simulink model "Model_15_11062020_3_Lev_Unbalance_SVM_AB21"  (R2021a)
settings: Solver=FixedStepAuto  StartTime=0.0  StopTime=0.03  FixedStep=Ts/10  MaxStep=1e-4  RelTol=1e-3
InitFcn:
  | Ts=1/(12000);
  | Ts_Control=Ts;
  | Ts_Power=Ts;
  | PulseDuration=5e-6;
  | Vrefpeak=399;
  | VDC=800;
  | R=1.4;
  | L=1e-4;
  | Freq = 120;
  | Rc= 0.00001;
  | C=220e-6;
  | Ld = 473e-6;
  | Lq = 1155e-6;
  | Fpm = 0.1383;
  | Rs = 0.036;
  | 
  | 
  | %%%%%Switch Characterization START%%%%%
  | T003_Thermal_Initialization;
  | T020_Characterizing_SKiM401MLI07E4_Simulink_Model_v1_0;
  | %%%%%Switch Characterization END%%%%%%
undefined symbols (not defined in the file or in its folder): Cond_Loss_Diode, Cond_Loss_IGBT, Page_Temp_C, Reverse_Rec_Diode, TurnoffIGBT, TurnonIGBT
libraries: spsMeanLib x35, simulink x28, spsMonostableLib x14, spsSampleandHoldLib x14, spsIGBTDiodeLib x12, spsDiodeLib x6, spsCurrentMeasurementLib x4, spsFirstOrderFilterLib x3, spsSeriesRLCBranchLib x3, spsVoltageMeasurementLib x3, pid_lib x2, spsAlphaBetaZerotoabcLib x1
(part 1 of 2)
settings Model: Creator=seoga  LastModifiedBy=Monster
settings SolverCC: AlgebraicLoopSolver=TrustRegion
settings DataIOCC: ReturnWorkspaceOutputs=off
settings DebuggingCC: SFMachineParentedDataDiag=warning  ArithmeticOperatorsInVariantConditions=warning
settings SFSimCC: SimUseLocalCustomCode=off  CustomCodeUndefinedFunction=UseInterfaceOnly
settings RTWCC: RTWUseLocalCustomCode=off

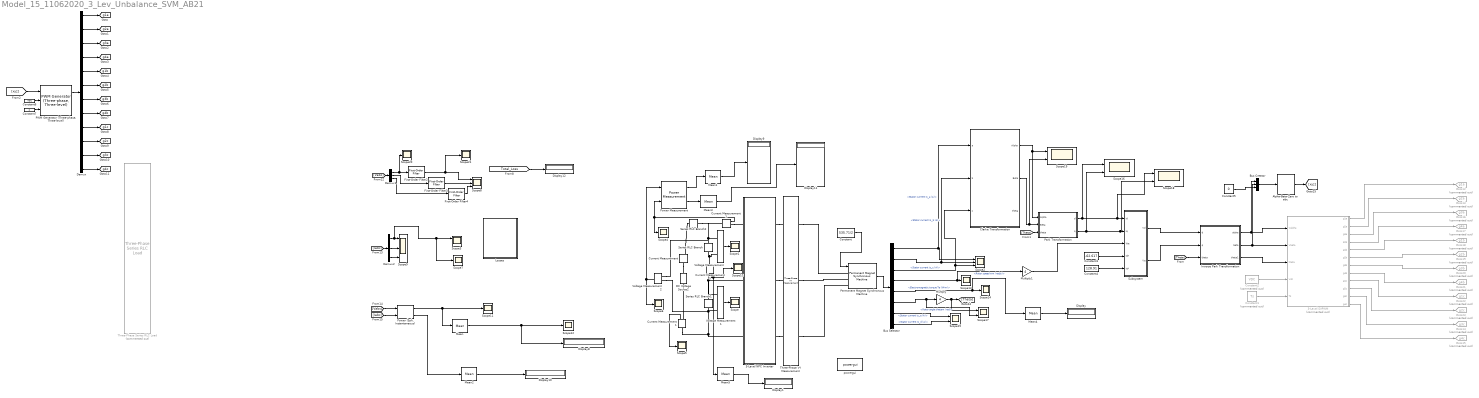
== system Model_15_11062020_3_Lev_Unbalance_SVM_AB21 ==
  3-Level NPC Inverter : Subsystem
  3-Level SVPWM : Subsystem  Commented=on
  Alpha-Beta-Zero to abc : spsAlphaBetaZerotoabcLib/Alpha-Beta-Zero to abc
      settings: SourceProductBaseCode=PS
  Bus Creator : BusCreator  Inputs=3
  Bus Selector : BusSelector  OutputSignals=Stator current is_a (A),Stator current is_b (A),Stator current is_c (A),Rotor speed wm (rad/s),Electromagnetic torque Te (N*m),Rotor angle thetam (rad),Stator current is_q (A),Stator current is_d (A)
  Clarke Transformation : Subsystem
  Constant : Constant  Value=535.71/2
  Constant1 : Constant  Commented=on  Value=Ts
  Constant2 : Constant  Commented=on  Value=VDC
  Constant3 : Constant  Value=-62.617
  Constant4 : Constant  Value=128.91
  Constant5 : Constant  Value=0
  Constant6 : Constant  Value=VDC
  Constant7 : Constant  Value=0
  Current Measurement{,1..3} (4 alike) : spsCurrentMeasurementLib/Current Measurement  PhasorSimulation=off  OutputType=Complex  PSBequivalent=0
  DC Voltage Source2 : spsDCVoltageSourceLib/DC Voltage Source  Amplitude=VDC  Measurements=None
  Demux : Demux  Outputs=12
  Demux1 : Demux  Outputs=3
  Demux2 : Demux  Outputs=3
  Display{,1,8..12} (7 alike) : Display
  First-Order Filter2 : spsFirstOrderFilterLib/First-Order Filter  FilterType=Lowpass  Tc=1e-4*2.5  Ts=0  Initialize=on  Vac_Init=[0, 0, 350/4]  Vdc_Init=0  PlotResponse=off  FreqRange="[0,  200,  1]"
  First-Order Filter3 : spsFirstOrderFilterLib/First-Order Filter  FilterType=Lowpass  Tc=1e-4  Ts=0  Initialize=on  Vac_Init=[0, 0, 350]  Vdc_Init=0  PlotResponse=off  FreqRange="[0,  200,  1]"
  First-Order Filter4 : spsFirstOrderFilterLib/First-Order Filter  FilterType=Lowpass  Tc=1e-4  Ts=0  Initialize=on  Vac_Init=[0, 0, 350]  Vdc_Init=0  PlotResponse=off  FreqRange="[0,  200,  1]"
  Goto12 : Goto  Commented=on  GotoTag=g1a  TagVisibility=global
  Goto13 : Goto  Commented=on  GotoTag=g2a  TagVisibility=global
  Goto14 : Goto  Commented=on  GotoTag=g3c  TagVisibility=global
  Goto15 : Goto  Commented=on  GotoTag=g4c  TagVisibility=global
  Goto16 : Goto  Commented=on  GotoTag=g3a  TagVisibility=global
  Goto17 : Goto  Commented=on  GotoTag=g4a  TagVisibility=global
  Goto18 : Goto  Commented=on  GotoTag=g1b  TagVisibility=global
  Goto19 : Goto  Commented=on  GotoTag=g2b  TagVisibility=global
  Goto20 : Goto  Commented=on  GotoTag=g3b  TagVisibility=global
  Goto21 : Goto  Commented=on  GotoTag=g4b  TagVisibility=global
  Goto22 : Goto  Commented=on  GotoTag=g1c  TagVisibility=global
  Goto23 : Goto  Commented=on  GotoTag=g2c  TagVisibility=global
  Inverse Park Transformation : Subsystem
  Losses : Subsystem
  Mean{,1..3} (4 alike) : spsMeanLib/Mean  Freq=Freq  Vinit=0  Ts=0
  Mean4 : spsMeanLib/Mean  Freq=1200  Vinit=0  Ts=0
  Mean5 : spsMeanLib/Mean  Freq=10  Vinit=0  Ts=0
  Multiply : Gain  Gain=4
  Multiply1 : Gain  Gain=4
  "PWM Generator (Three-phase, Three-level)" : eePwmGeneratorThreeLevel/PWM Generator (Three-phase, Three-level)  CPWMMode=SVM: space vector modulation  fsw=1/Ts  Ts=Ts/10
      settings: SourceProductBaseCode=PS  SamplingMode=Natural
  Park Transformation : Subsystem
  Permanent Magnet Synchronous Machine : spsPermanentMagnetSynchronousMachineLib/Permanent Magnet Synchronous Machine  NbPhases=3  FluxDistribution=Sinusoidal  RotorType=Salient-pole  MechanicalLoad=Speed w  PresetModel=No  ShowDetailedParameters=on  MeasurementBus=off  Resistance=0.036  Inductance=8.5e-3  dqInductances=[0.473e-3,1.155e-3]  La=0.000395  MachineConstant=Flux linkage established by magnets (V.s)  Flux=0.1383  VoltageCst=100.3394  TorqueCst=0.8298  Flat=120  Mechanical=[0.0027 0.0004924 4 0]  PolePairs=4  InitialConditions=[0,0, 0,0]  InitialConditions5ph=[0 0 0 0 0 0]  RefAngle=Aligned with phase A axis (original Park)  IterativeDiscreteModel=Trapezoidal non iterative  TsBlock=-1  TsPowergui=0
  "Power (3ph, Instantaneous)" : spsPower3phInstantaneousLib/Power (3ph, Instantaneous)
  Power Measurement : eePowerMeasurement/Power Measurement  LabelModeActiveChoice=Continuous  F=60  K=[0 1 2 3]  Ts=0
      settings: SourceProductBaseCode=PS
  Scope{,1,4..7,10..14,20..21} (13 alike) : Scope
  Scope{3,15..19} (6 alike) : Scope  NumInputPorts=2
  Scope2 : Scope  NumInputPorts=3
  Scope8 : Scope  NumInputPorts=3
  Scope9 : Scope  NumInputPorts=3
  Series RLC Branch : spsSeriesRLCBranchLib/Series RLC Branch  LConnTagsString=__new0  RConnTagsString=__new0  BranchType=RC  Resistance=Rc  Inductance=1e-3  SetiL0=off  InitialCurrent=0  Capacitance=C  Setx0=on  InitialVoltage=VDC/2  Measurements=None
  Series RLC Branch1 : spsSeriesRLCBranchLib/Series RLC Branch  LConnTagsString=__new0  RConnTagsString=__new0  BranchType=RC  Resistance=Rc  Inductance=1e-3  SetiL0=off  InitialCurrent=0  Capacitance=C  Setx0=on  InitialVoltage=VDC/2  Measurements=None
  Series RLC Branch2 : spsSeriesRLCBranchLib/Series RLC Branch  LConnTagsString=__new0  RConnTagsString=__new0  BranchType=R  Resistance=1e-6  Inductance=1e-3  SetiL0=off  InitialCurrent=0  Capacitance=470e-6  Setx0=on  InitialVoltage=400  Measurements=None
  Subsystem : Subsystem
  Three-Phase Series RLC Load : spsThreePhaseSeriesRLCLoadLib/Three-Phase Series RLC Load  Commented=on  LConnTagsString=A|B|C  Configuration=Y (grounded)  NominalVoltage=Vrefpeak*sqrt(3/2)  Vabc=[1e3 1e3 1e3]  Vabcp=[1e3 1e3 1e3]  NominalFrequency=Freq  UnbalancedPower=off  ActivePower=150e3  InductivePower=100e3  CapacitivePower=0  Pabc=[10e3 9e3 11e3]  QLabc=[100 90 110]  QCabc=[100 90 110]  Pabcp=[10e3 9e3 11e3]  QLabcp=[100 90 110]  QCabcp=[100 90 110]  Measurements=None  LoadType=constant Z
  Three-Phase V-I Measurement : spsThreePhaseVIMeasurementLib/Three-Phase V-I Measurement  VoltageMeasurement=phase-to-phase  SetLabelV=on  LabelV=Vabc  Vpu=off  VpuLL=off  CurrentMeasurement=yes  SetLabelI=on  LabelI=Iabc  Ipu=off  Pbase=100e6  Vbase=500e3  OutputType=Complex  PhasorSimulation=off  PSBequivalent=0
  Voltage Measurement : spsVoltageMeasurementLib/Voltage Measurement  PhasorSimulation=off  OutputType=Complex  PSBequivalent=0
  Voltage Measurement1 : spsVoltageMeasurementLib/Voltage Measurement  PhasorSimulation=off  OutputType=Complex  PSBequivalent=0
  Voltage Measurement2 : spsVoltageMeasurementLib/Voltage Measurement  PhasorSimulation=off  OutputType=Complex  PSBequivalent=0
  powergui : spspowerguiLib/powergui  Priority=1  SimulationMode=Discrete  SampleTime=Ts/10  frequency=60  Iterations=50  frequencyindice=0  Pbase=100e6  ErrMax=1e-4  UnitsV=kV  UnitsW=MW  buscounter=0  FunctionMessages=off  echomessages=off  EnableUseOfTLC=off  CurrentSourceSwitches=off  DisableSnubberDevices=off  DisableRonSwitches=off  DisableVfSwitches=off  DisplayEquations=off  AutomaticDiscreteSolvers=off  SolverType=Tustin/Backward Euler (TBE)  Interpol=off  ExternalGateDelay=off  methode=off  Ts=100  x0status=blocks  SPID=off  SwTol=0  HookPort=off  NonlinearTolerance=1e-4  nMaxIteration=100  ContinueOnMaxIteration=off  RestoreLinks=warning  ResistiveCurrentMeasurement=off  Frange=[0:2:500]  Ylog=off  Xlog=on  ShowGrid=off  save=off  variable=ZData  structure=0  ZoomFFT=off  StartTime=0.0  cycles=1  DisplayStyle=1  fundamental=60  FreqAxis=off  MaxFrequency=1000  frequencyindicesteady=1  RmsSteady=1  display=off
  tag scope: g1a=global, g1b=global, g1c=global, g2a=global, g2b=global, g2c=global, g3a=global, g3b=global, g3c=global, g4a=global, g4b=global, g4c=global
  wires:
  Bus Selector/2 -> Clarke Transformation/2(b), Scope2/2  "<Stator current is_b (A)>"
  Demux1/3 -> First-Order Filter4/1
  "Power (3ph, Instantaneous)"/1 -> Mean/1, Scope11/1
  [Vabc] -> Demux1/1
  Demux1/2 -> First-Order Filter3/1
  First-Order Filter4/1 -> Scope8/3
  [Vabc] -> "Power (3ph, Instantaneous)"/1
  Demux1/1 -> Scope20/1, First-Order Filter2/1
  [Iabc] -> Demux2/1
  [Iabc] -> "Power (3ph, Instantaneous)"/2
  First-Order Filter3/1 -> Scope8/2
  Voltage Measurement1/1 -> Scope/1
  Voltage Measurement/1 -> Scope1/1
  Constant7/1 -> "PWM Generator (Three-phase, Three-level)"/3
  Constant6/1 -> "PWM Generator (Three-phase, Three-level)"/2
  Demux/10 -> [g2c]
  Demux/3 -> [g3a]
  Demux/4 -> [g4a]
  Demux/7 -> [g3b]
  Demux/8 -> [g4b]
  Demux/5 -> [g1b]
  Demux/11 -> [g3c]
  Demux/6 -> [g2b]
  "PWM Generator (Three-phase, Three-level)"/1 -> Demux/1
  Demux/1 -> [g1a]
  Demux/2 -> [g2a]
  Demux/9 -> [g1c]
  Demux/12 -> [g4c]
  Mean/1 -> Display8/1, Scope12/1
  Mean2/1 -> Display10/1
  "Power (3ph, Instantaneous)"/2 -> Mean2/1
  Demux2/1 -> Scope7/1, Scope3/1, Scope9/1
  Demux2/2 -> Scope9/2
  Demux2/3 -> Scope9/3
  Voltage Measurement2/1 -> Scope6/1, Power Measurement/1
  Power Measurement/1 -> Mean1/1
  Mean1/1 -> Display9/1
  Power Measurement/2 -> Mean3/1
  Mean3/1 -> Display11/1
  Current Measurement1/1 -> Scope5/1
  Current Measurement2/1 -> Scope4/1, Power Measurement/2
  [Total_Loss] -> Display12/1
  Current Measurement3/1 -> Mean5/1, Scope10/1
  Permanent Magnet Synchronous Machine/1 -> Bus Selector/1
  3-Level SVPWM/2(g2a) -> Goto13/1
  3-Level SVPWM/1(g1a) -> Goto12/1
  3-Level SVPWM/11(g3c) -> Goto14/1
  3-Level SVPWM/6(g2b) -> Goto19/1
  3-Level SVPWM/4(g4a) -> Goto17/1
  3-Level SVPWM/8(g4b) -> Goto21/1
  3-Level SVPWM/9(g1c) -> Goto22/1
  3-Level SVPWM/10(g2c) -> Goto23/1
  3-Level SVPWM/7(g3b) -> Goto20/1
  3-Level SVPWM/12(g4c) -> Goto15/1
  3-Level SVPWM/3(g3a) -> Goto16/1
  3-Level SVPWM/5(g1b) -> Goto18/1
  Inverse Park Transformation/1(alpha) -> Bus Creator/1, 3-Level SVPWM/1(Valpha)
  Inverse Park Transformation/2(beta) -> Bus Creator/2, 3-Level SVPWM/2(Vbeta)
  Inverse Park Transformation/3(theta1) -> 3-Level SVPWM/3(theta)
  Constant1/1 -> 3-Level SVPWM/5(Ts)
  Constant2/1 -> 3-Level SVPWM/4(Vdc)
  Bus Selector/1 -> Clarke Transformation/1(a), Scope2/1  "<Stator current is_a (A)>"
  Bus Selector/3 -> Clarke Transformation/3(c), Scope2/3  "<Stator current is_c (A)>"
  Bus Selector/4 -> Multiply1/1, Scope13/1  "<Rotor speed wm (rad/s)>"
  Bus Selector/5 -> Mean4/1, Scope14/1  "<Electromagnetic torque Te (N*m)>"
  Constant/1 -> Permanent Magnet Synchronous Machine/1
  [Theta] -> Inverse Park Transformation/3(theta)
  Clarke Transformation/1(Alpha) -> Scope19/1, Park Transformation/1(Alpha)
  Clarke Transformation/2(Beta) -> Scope19/2, Park Transformation/2(Beta)
  [Theta] -> Park Transformation/3(theta)
  Bus Selector/6 -> Scope17/2, Multiply/1  "<Rotor angle thetam (rad)>"
  Multiply/1 -> Scope17/1, [Theta]
  Multiply1/1 -> Subsystem/3(We)
  Constant4/1 -> Subsystem/5(Iq*)
  Constant3/1 -> Subsystem/4(Id*)
  Subsystem/2(Vq) -> Inverse Park Transformation/2(q)
  Subsystem/1(Vd) -> Inverse Park Transformation/1(d)
  Bus Selector/7 -> Scope15/1  "<Stator current is_q (A)>"
  Bus Selector/8 -> Scope15/2  "<Stator current is_d (A)>"
  Mean4/1 -> Display/1
  Mean5/1 -> Display1/1
  Park Transformation/1(d) -> Scope18/1, Subsystem/1(Id), Scope16/1
  Park Transformation/2(q) -> Scope18/2, Subsystem/2(Iq), Scope16/2
  Bus Creator/1 -> Alpha-Beta-Zero to abc/1
  [xyz] -> "PWM Generator (Three-phase, Three-level)"/1
  Alpha-Beta-Zero to abc/1 -> [xyz]
  Constant5/1 -> Bus Creator/3
  First-Order Filter2/1 -> Scope21/1, Scope8/1
  connections:
  Series RLC Branch/LConn1 -- Series RLC Branch2/RConn1 -- Current Measurement2/LConn1 -- Voltage Measurement2/LConn1 -- Voltage Measurement/LConn1
  Series RLC Branch/RConn1 -- Current Measurement3/LConn1 -- Voltage Measurement/LConn2
  Series RLC Branch1/RConn1 -- Voltage Measurement2/LConn2 -- Voltage Measurement1/LConn2 -- Current Measurement1/LConn1 -- 3-Level NPC Inverter/LConn3
  Current Measurement/RConn1 -- Series RLC Branch2/LConn1
  Current Measurement/LConn1 -- DC Voltage Source2/RConn1
  Current Measurement1/RConn1 -- DC Voltage Source2/LConn1
  Current Measurement2/RConn1 -- 3-Level NPC Inverter/LConn1
  Series RLC Branch1/LConn1 -- Voltage Measurement1/LConn1 -- Current Measurement3/RConn1 -- 3-Level NPC Inverter/LConn2
  3-Level NPC Inverter/RConn1 -- Three-Phase V-I Measurement/LConn1
  Three-Phase V-I Measurement/RConn1 -- Permanent Magnet Synchronous Machine/LConn1
  Three-Phase V-I Measurement/RConn2 -- Permanent Magnet Synchronous Machine/LConn2
  3-Level NPC Inverter/RConn2 -- Three-Phase V-I Measurement/LConn2
  Three-Phase V-I Measurement/RConn3 -- Permanent Magnet Synchronous Machine/LConn3
  3-Level NPC Inverter/RConn3 -- Three-Phase V-I Measurement/LConn3

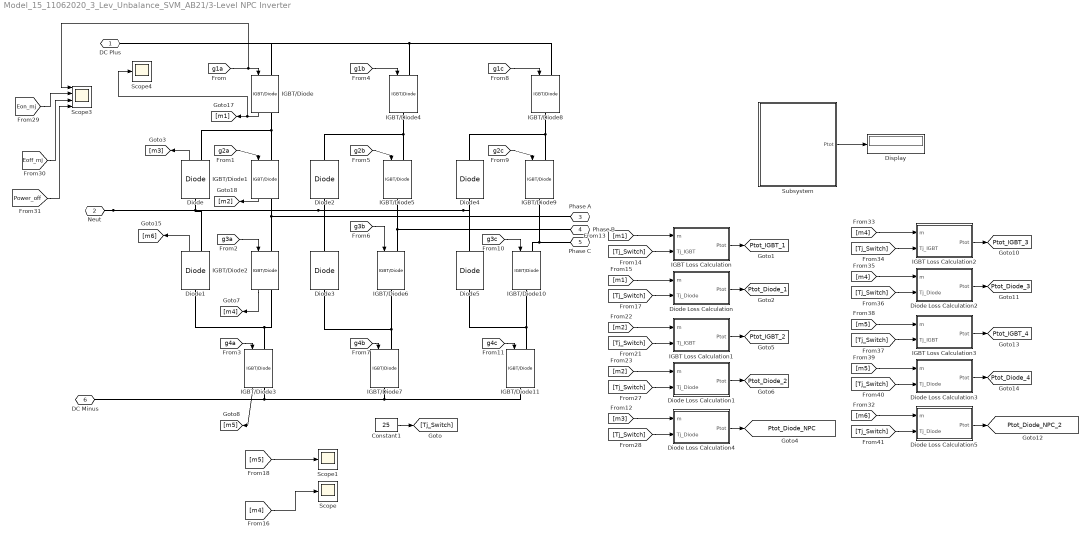
== system Model_15_11062020_3_Lev_Unbalance_SVM_AB21/3-Level NPC Inverter ==
  Constant1 : Constant  Value=25
  Diode : spsDiodeLib/Diode  Ron=1e-5  Lon=0  Vf=0.8  IC=0  UseSnubber=0  Rs=1e6  Cs=inf  Measurements=on
  Diode Loss Calculation : Subsystem
  Diode Loss Calculation1 : Subsystem
  Diode Loss Calculation2 : Subsystem
  Diode Loss Calculation3 : Subsystem
  Diode Loss Calculation4 : Subsystem
  Diode Loss Calculation5 : Subsystem
  Diode1 : spsDiodeLib/Diode  Ron=1e-5  Lon=0  Vf=0.8  IC=0  UseSnubber=0  Rs=1e6  Cs=inf  Measurements=on
  Diode{2..5} (4 alike) : spsDiodeLib/Diode  Ron=1e-5  Lon=0  Vf=0.8  IC=0  UseSnubber=0  Rs=1e6  Cs=inf  Measurements=off
  Display : Display
  IGBT Loss Calculation : Subsystem
  IGBT Loss Calculation1 : Subsystem
  IGBT Loss Calculation2 : Subsystem
  IGBT Loss Calculation3 : Subsystem
  IGBT/Diode{,1..3} (4 alike) : spsIGBTDiodeLib/IGBT//Diode  Ron=1e-3  Rs=1e6  Cs=inf  Measurements=on
  IGBT/Diode{4..11} (8 alike) : spsIGBTDiodeLib/IGBT//Diode  Ron=1e-3  Rs=1e6  Cs=inf  Measurements=off
  Scope : Scope
  Scope1 : Scope
  Scope3 : Scope  NumInputPorts=4
  Scope4 : Scope
  Subsystem : Subsystem
  DC Plus : PMIOPort  Side=Left
  " Neut" : PMIOPort  Port=2  Side=Left
  Phase A : PMIOPort  Port=3  Side=Right
  Phase B : PMIOPort  Port=4  Side=Right
  Phase C : PMIOPort  Port=5  Side=Right
  DC Minus : PMIOPort  Port=6  Side=Left
  tag scope: Ptot_Diode_1=global, Ptot_Diode_2=global, Ptot_Diode_3=global, Ptot_Diode_4=global, Ptot_Diode_NPC=global, Ptot_Diode_NPC_2=global, Ptot_IGBT_1=global, Ptot_IGBT_2=global, Ptot_IGBT_3=global, Ptot_IGBT_4=global
  wires:
  [g1a] -> Scope3/1, IGBT/Diode/1
  [g3a] -> IGBT/Diode2/1
  [g2b] -> IGBT/Diode5/1
  [g3b] -> IGBT/Diode6/1
  [g4b] -> IGBT/Diode7/1
  [g2c] -> IGBT/Diode9/1
  [g3c] -> IGBT/Diode10/1
  [g4c] -> IGBT/Diode11/1
  [g4a] -> IGBT/Diode3/1
  [g1b] -> IGBT/Diode4/1
  [g1c] -> IGBT/Diode8/1
  [g2a] -> IGBT/Diode1/1
  IGBT Loss Calculation/1(Ptot) -> [Ptot_IGBT_1]
  [m1] -> IGBT Loss Calculation/1(m)
  [m1] -> Diode Loss Calculation/1(m)
  Diode Loss Calculation/1(Ptot) -> [Ptot_Diode_1]
  IGBT Loss Calculation1/1(Ptot) -> [Ptot_IGBT_2]
  Diode Loss Calculation1/1(Ptot) -> [Ptot_Diode_2]
  [m2] -> Diode Loss Calculation1/1(m)
  [m2] -> IGBT Loss Calculation1/1(m)
  IGBT/Diode/1 -> Scope4/1, [m1]
  IGBT/Diode1/1 -> [m2]
  Diode/1 -> [m3]
  Diode Loss Calculation4/1(Ptot) -> [Ptot_Diode_NPC]
  [m3] -> Diode Loss Calculation4/1(m)
  Constant1/1 -> [Tj_Switch]
  [Tj_Switch] -> IGBT Loss Calculation/2(Tj_IGBT)
  [Tj_Switch] -> Diode Loss Calculation/2(Tj_Diode)
  [Tj_Switch] -> IGBT Loss Calculation1/2(Tj_IGBT)
  [Tj_Switch] -> Diode Loss Calculation1/2(Tj_Diode)
  [Tj_Switch] -> Diode Loss Calculation4/2(Tj_Diode)
  IGBT/Diode2/1 -> [m4]
  [m4] -> Scope/1
  IGBT/Diode3/1 -> [m5]
  [m5] -> Scope1/1
  [Eon_mj] -> Scope3/2
  [Eoff_mj] -> Scope3/3
  [Power_off] -> Scope3/4
  [m4] -> Diode Loss Calculation2/1(m)
  Diode Loss Calculation5/1(Ptot) -> [Ptot_Diode_NPC_2]
  [m5] -> Diode Loss Calculation3/1(m)
  [Tj_Switch] -> Diode Loss Calculation3/2(Tj_Diode)
  [m5] -> IGBT Loss Calculation3/1(m)
  [m6] -> Diode Loss Calculation5/1(m)
  [Tj_Switch] -> Diode Loss Calculation5/2(Tj_Diode)
  IGBT Loss Calculation3/1(Ptot) -> [Ptot_IGBT_4]
  [Tj_Switch] -> IGBT Loss Calculation2/2(Tj_IGBT)
  Diode Loss Calculation2/1(Ptot) -> [Ptot_Diode_3]
  Diode Loss Calculation3/1(Ptot) -> [Ptot_Diode_4]
  [Tj_Switch] -> Diode Loss Calculation2/2(Tj_Diode)
  [m4] -> IGBT Loss Calculation2/1(m)
  [Tj_Switch] -> IGBT Loss Calculation3/2(Tj_IGBT)
  IGBT Loss Calculation2/1(Ptot) -> [Ptot_IGBT_3]
  Diode1/1 -> [m6]
  Subsystem/1(Ptot) -> Display/1
  connections:
  IGBT/Diode11/RConn1 -- IGBT/Diode7/RConn1 -- DC Minus/RConn1 -- IGBT/Diode3/RConn1
  IGBT/Diode1/LConn1 -- IGBT/Diode/RConn1 -- Diode/RConn1
  IGBT/Diode9/RConn1 -- Phase C/RConn1 -- IGBT/Diode10/LConn1
  IGBT/Diode5/RConn1 -- Phase B/RConn1 -- IGBT/Diode6/LConn1
  IGBT/Diode11/LConn1 -- Diode5/LConn1 -- IGBT/Diode10/RConn1
  IGBT/Diode7/LConn1 -- Diode3/LConn1 -- IGBT/Diode6/RConn1
  IGBT/Diode1/RConn1 -- Phase A/RConn1 -- IGBT/Diode2/LConn1
  IGBT/Diode5/LConn1 -- Diode2/RConn1 -- IGBT/Diode4/RConn1
  IGBT/Diode3/LConn1 -- Diode1/LConn1 -- IGBT/Diode2/RConn1
  IGBT/Diode9/LConn1 -- Diode4/RConn1 -- IGBT/Diode8/RConn1
  " Neut"/RConn1 -- Diode1/RConn1 -- Diode3/RConn1 -- Diode2/LConn1 -- Diode5/RConn1 -- Diode4/LConn1 -- Diode/LConn1
  IGBT/Diode8/LConn1 -- IGBT/Diode/LConn1 -- DC Plus/RConn1 -- IGBT/Diode4/LConn1

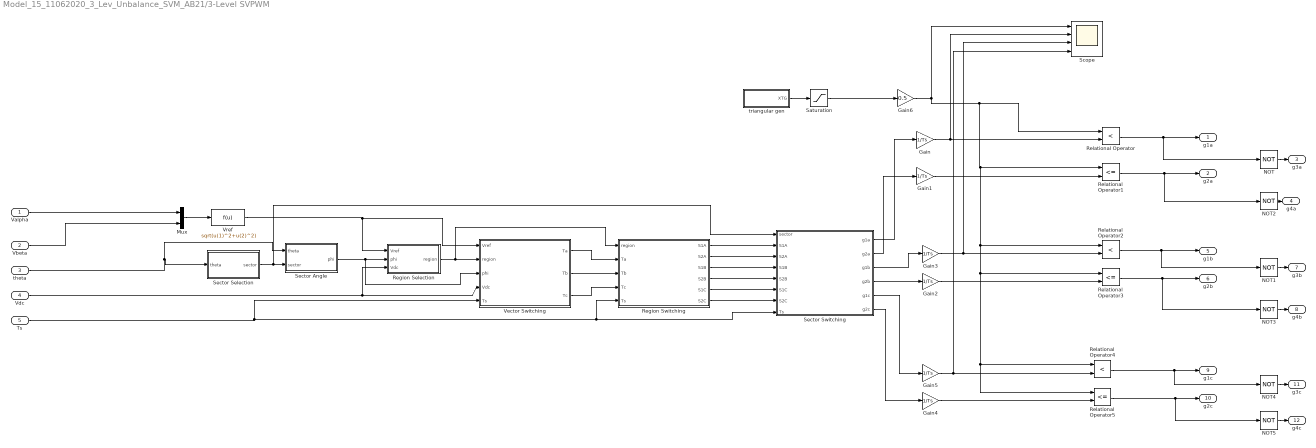
== system Model_15_11062020_3_Lev_Unbalance_SVM_AB21/3-Level SVPWM ==
  Valpha : Inport
  Vbeta : Inport  Port=2
  theta : Inport  Port=3
  Vdc : Inport  Port=4
  Ts : Inport  Port=5
  Gain{,1..5} (6 alike) : Gain  Gain=1/Ts
  Gain6 : Gain  Gain=0.5
  Mux : Mux  Inputs=2
  NOT{,1..5} (6 alike) : Logic  Operator=NOT  IconShape=distinctive  AllPortsSameDT=off  OutDataTypeStr=boolean
  Region Selection : MATLAB Function  TreatAsAtomicUnit=on
  Region Switching : MATLAB Function  TreatAsAtomicUnit=on
  Relational Operator : RelationalOperator  Operator=<  OutDataTypeStr=boolean  RndMeth=Nearest
  Relational Operator1 : RelationalOperator  Operator=<=  OutDataTypeStr=boolean  RndMeth=Nearest
  Relational Operator2 : RelationalOperator  Operator=<  OutDataTypeStr=boolean  RndMeth=Nearest
  Relational Operator3 : RelationalOperator  Operator=<=  OutDataTypeStr=boolean  RndMeth=Nearest
  Relational Operator4 : RelationalOperator  Operator=<  OutDataTypeStr=boolean  RndMeth=Nearest
  Relational Operator5 : RelationalOperator  Operator=<=  OutDataTypeStr=boolean  RndMeth=Nearest
  Saturation : Saturate  UpperLimit=1  LowerLimit=0
  Scope : Scope  NumInputPorts=4
  Sector Angle : MATLAB Function  TreatAsAtomicUnit=on
  Sector Selection : MATLAB Function  TreatAsAtomicUnit=on
  Sector Switching : MATLAB Function  TreatAsAtomicUnit=on
  Vector Switching : MATLAB Function  TreatAsAtomicUnit=on
  Vref : Fcn  Expr=sqrt(u(1)^2+u(2)^2)
  triangular gen : Subsystem
  g1a : Outport
  g2a : Outport  Port=2
  g3a : Outport  Port=3
  g4a : Outport  Port=4
  g1b : Outport  Port=5
  g2b : Outport  Port=6
  g3b : Outport  Port=7
  g4b : Outport  Port=8
  g1c : Outport  Port=9
  g2c : Outport  Port=10
  g3c : Outport  Port=11
  g4c : Outport  Port=12
  wires:
  Mux/1 -> Vref/1
  theta/1 -> Sector Angle/1(theta), Sector Selection/1(theta)
  Sector Angle/1(phi) -> Vector Switching/3(phi), Region Selection/2(phi)
  Vref/1 -> Vector Switching/1(Vref), Region Selection/1(Vref)
  Vdc/1 -> Region Selection/3(Vdc), Vector Switching/4(Vdc)
  Region Selection/1(region) -> Vector Switching/2(region), Region Switching/1(region)
  Vector Switching/3(Tc) -> Region Switching/4(Tc)
  Vector Switching/2(Tb) -> Region Switching/3(Tb)
  Vector Switching/1(Ta) -> Region Switching/2(Ta)
  Region Switching/1(S1A) -> Sector Switching/2(S1A)
  Region Switching/2(S2A) -> Sector Switching/3(S2A)
  Region Switching/3(S1B) -> Sector Switching/4(S1B)
  Region Switching/4(S2B) -> Sector Switching/5(S2B)
  Region Switching/5(S1C) -> Sector Switching/6(S1C)
  Region Switching/6(S2C) -> Sector Switching/7(S2C)
  Sector Selection/1(sector) -> Sector Angle/2(sector), Sector Switching/1(sector)
  NOT/1 -> g3a/1
  NOT1/1 -> g3b/1
  NOT2/1 -> g4a/1
  NOT3/1 -> g4b/1
  NOT5/1 -> g4c/1
  NOT4/1 -> g3c/1
  Sector Switching/1(g1a) -> Gain/1
  Sector Switching/3(g1b) -> Gain3/1
  Sector Switching/5(g1c) -> Gain5/1
  Sector Switching/4(g2b) -> Gain2/1
  Sector Switching/2(g2a) -> Gain1/1
  Sector Switching/6(g2c) -> Gain4/1
  Gain/1 -> Scope/2, Relational Operator/2
  Relational Operator/1 -> NOT/1, g1a/1
  Gain1/1 -> Relational Operator1/2
  Gain5/1 -> Scope/4, Relational Operator4/2
  Gain4/1 -> Relational Operator5/2
  Gain2/1 -> Relational Operator3/2
  Gain3/1 -> Scope/3, Relational Operator2/2
  Relational Operator1/1 -> NOT2/1, g2a/1
  Relational Operator2/1 -> NOT1/1, g1b/1
  Relational Operator3/1 -> NOT3/1, g2b/1
  Relational Operator4/1 -> NOT4/1, g1c/1
  Relational Operator5/1 -> NOT5/1, g2c/1
  Valpha/1 -> Mux/1
  Vbeta/1 -> Mux/2
  Ts/1 -> Sector Switching/8(Ts), Region Switching/5(Ts), Vector Switching/5(Ts)
  triangular gen/1(XTG) -> Saturation/1
  Gain6/1 -> Scope/1, Relational Operator3/1, Relational Operator5/1, Relational Operator4/1, Relational Operator2/1, Relational Operator1/1, Relational Operator/1
  Saturation/1 -> Gain6/1

== system Model_15_11062020_3_Lev_Unbalance_SVM_AB21/Clarke Transformation ==
  a : Inport
  b : Inport  Port=2
  c : Inport  Port=3
  AlphaTransformation : Sum  Inputs=|+--
  Alpha_Gain : Gain  Gain=2/3
  Beta Transformation : Sum  Inputs=|+-
  Beta_Gain : Gain  Gain=2/3
  Gain1 : Gain  Gain=0.5
  Gain2 : Gain  Gain=0.5
  Gain3 : Gain  Gain=sqrt(3)/2
  Gain4 : Gain  Gain=sqrt(3)/2
  Trigonometric Function : Trigonometry  Operator=atan2
  Alpha : Outport
  Beta : Outport  Port=2
  theta : Outport  Port=3
  wires:
  Gain1/1 -> AlphaTransformation/2
  Gain4/1 -> Beta Transformation/2
  AlphaTransformation/1 -> Alpha_Gain/1
  Gain3/1 -> Beta Transformation/1
  b/1 -> Gain1/1, Gain3/1
  Gain2/1 -> AlphaTransformation/3
  c/1 -> Gain2/1, Gain4/1
  Beta Transformation/1 -> Beta_Gain/1
  a/1 -> AlphaTransformation/1
  Trigonometric Function/1 -> theta/1
  Alpha_Gain/1 -> Trigonometric Function/2, Alpha/1
  Beta_Gain/1 -> Trigonometric Function/1, Beta/1

== system Model_15_11062020_3_Lev_Unbalance_SVM_AB21/Inverse Park Transformation ==
  d : Inport
  q : Inport  Port=2
  theta : Inport  Port=3
  Product{,1..3} (4 alike) : Product
  Sum : Sum  Inputs=|+-
  Sum1 : Sum  Inputs=|++
  Trigonometric Function : Trigonometry
  Trigonometric Function1 : Trigonometry  Operator=cos
  Trigonometric Function2 : Trigonometry  Operator=atan2
  alpha : Outport
  beta : Outport  Port=2
  theta1 : Outport  Port=3
  wires:
  Product/1 -> Sum1/1
  Trigonometric Function/1 -> Product1/2, Product/2
  d/1 -> Product2/1, Product/1
  Product2/1 -> Sum/1
  theta/1 -> Trigonometric Function/1, Trigonometric Function1/1
  Product1/1 -> Sum/2
  Trigonometric Function1/1 -> Product2/2, Product3/2
  q/1 -> Product3/1, Product1/1
  Product3/1 -> Sum1/2
  Sum/1 -> Trigonometric Function2/2, alpha/1
  Trigonometric Function2/1 -> theta1/1
  Sum1/1 -> Trigonometric Function2/1, beta/1

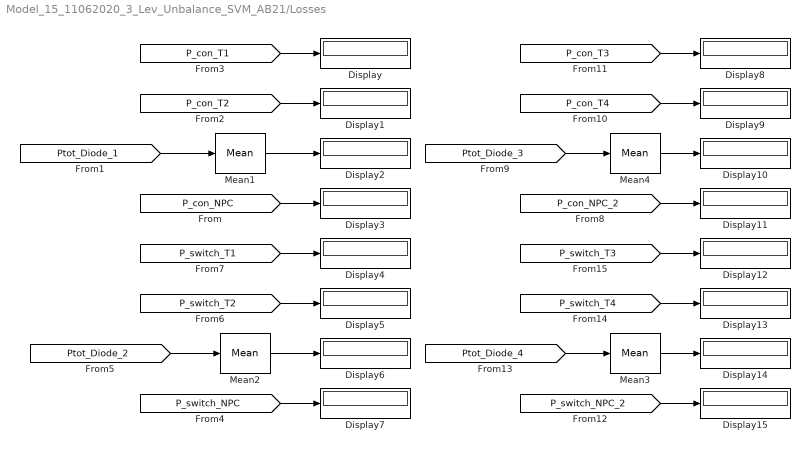
== system Model_15_11062020_3_Lev_Unbalance_SVM_AB21/Losses ==
  Display{,1..15} (16 alike) : Display
  Mean{1..4} (4 alike) : spsMeanLib/Mean  Freq=Freq  Vinit=0  Ts=0
  wires:
  [P_con_T1] -> Display/1
  [P_switch_T2] -> Display5/1
  [P_switch_T1] -> Display4/1
  [P_switch_NPC] -> Display7/1
  [P_con_NPC] -> Display3/1
  [P_con_T2] -> Display1/1
  [P_con_T4] -> Display9/1
  [P_con_T3] -> Display8/1
  [P_switch_T3] -> Display12/1
  [P_con_NPC_2] -> Display11/1
  [P_switch_T4] -> Display13/1
  [P_switch_NPC_2] -> Display15/1
  [Ptot_Diode_2] -> Mean2/1
  Mean2/1 -> Display6/1
  [Ptot_Diode_1] -> Mean1/1
  Mean1/1 -> Display2/1
  [Ptot_Diode_4] -> Mean3/1
  Mean3/1 -> Display14/1
  [Ptot_Diode_3] -> Mean4/1
  Mean4/1 -> Display10/1

== system Model_15_11062020_3_Lev_Unbalance_SVM_AB21/Park Transformation ==
  Alpha : Inport
  Beta : Inport  Port=2
  theta : Inport  Port=3
  Product{,1..3} (4 alike) : Product
  Trigonometric Function1 : Trigonometry
  Trigonometric Function2 : Trigonometry  Operator=cos
  d_sum : Sum  Inputs=|++
  q_sum : Sum  Inputs=|-+
  d : Outport
  q : Outport  Port=2
  wires:
  Trigonometric Function1/1 -> Product2/2, Product1/2
  Product/1 -> d_sum/1
  Product2/1 -> q_sum/1
  Beta/1 -> Product3/1, Product1/1
  Alpha/1 -> Product2/1, Product/1
  Product3/1 -> q_sum/2
  Trigonometric Function2/1 -> Product3/2, Product/2
  Product1/1 -> d_sum/2
  q_sum/1 -> q/1
  d_sum/1 -> d/1
  theta/1 -> Trigonometric Function2/1, Trigonometric Function1/1

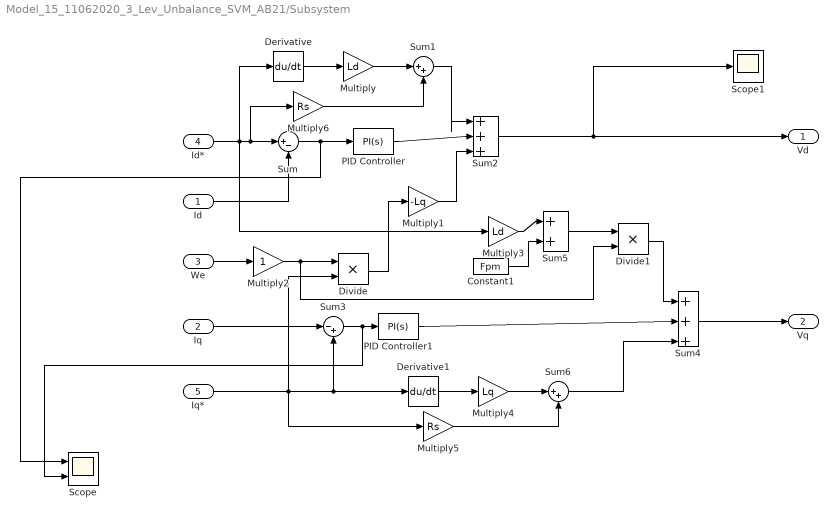
== system Model_15_11062020_3_Lev_Unbalance_SVM_AB21/Subsystem ==
  Id : Inport
  Iq : Inport  Port=2
  We : Inport  Port=3
  Id* : Inport  Port=4
  Iq* : Inport  Port=5
  Constant1 : Constant  Value=Fpm
  Derivative : Derivative
  Derivative1 : Derivative
  Divide : Product  Inputs=**
  Divide1 : Product  Inputs=**
  Multiply : Gain  Gain=Ld
  Multiply1 : Gain  Gain=-Lq
  Multiply2 : Gain
  Multiply3 : Gain  Gain=Ld
  Multiply4 : Gain  Gain=Lq
  Multiply5 : Gain  Gain=Rs
  Multiply6 : Gain  Gain=Rs
  PID Controller : pid_lib/PID Controller  Controller=PI  Form=Parallel  TimeDomain=Continuous-time  UseExternalTs=off  SampleTime=-1  IntegratorMethod=Forward Euler  FilterMethod=Forward Euler  ControllerParametersSource=internal  P=0.2  I=0.1  D=0  UseFilter=on  N=100  TunerSelectOption=Transfer Function Based (PID Tuner App)  InitialConditionSource=internal  InitialConditionForIntegrator=0  InitialConditionForFilter=0  DifferentiatorICPrevScaledInput=0  ExternalReset=none  TrackingMode=off  Kt=1  LimitOutput=off  SatLimitsSource=internal  UpperSaturationLimit=inf  LowerSaturationLimit=-inf  LinearizeAsGain=on  AntiWindupMode=none  Kb=1  POutMin=[]  POutMax=[]  IOutMin=[]  IOutMax=[]  DOutMin=[]  DOutMax=[]  NOutMin=[]  NOutMax=[]  SumOutMin=[]  SumOutMax=[]  SaturationOutMin=[]  SaturationOutMax=[]  PParamMin=[]  PParamMax=[]  IParamMin=[]  IParamMax=[]  DParamMin=[]  DParamMax=[]  NParamMin=[]  NParamMax=[]  KbParamMin=[]  KbParamMax=[]  KtParamMin=[]  KtParamMax=[]  KbOutMin=[]  KbOutMax=[]  KtOutMin=[]  KtOutMax=[]  IntegratorOutMin=[]  IntegratorOutMax=[]  FilterOutMin=[]  FilterOutMax=[]  SumI1OutMin=[]  SumI1OutMax=[]  SumI2OutMin=[]  SumI2OutMax=[]  SumI3OutMin=[]  SumI3OutMax=[]  SumI4OutMin=[]  SumI4OutMax=[]  SumDOutMin=[]  SumDOutMax=[]  DifferentiatorOutMin=[]  DifferentiatorOutMax=[]  FilterDiffOutCoefMin=[]  FilterDiffOutCoefMax=[]  ReciprocalOutMin=[]  ReciprocalOutMax=[]  SumDenOutMin=[]  SumDenOutMax=[]  SumNumOutMin=[]  SumNumOutMax=[]  DivideOutMin=[]  DivideOutMax=[]  UdiffTsProdOutMin=[]  UdiffTsProdOutMax=[]  NTsProdOutMin=[]  NTsProdOutMax=[]  UintegralTsProdOutMin=[]  UintegralTsProdOutMax=[]  UngainTsProdOutMin=[]  UngainTsProdOutMax=[]  IntegratorContinuousStateAttributes=''  IntegratorStateMustResolveToSignalObject=off  IntegratorRTWStateStorageClass=Auto  FilterContinuousStateAttributes=''  FilterStateMustResolveToSignalObject=off  FilterRTWStateStorageClass=Auto  ParallelPVariant=InternalParameters  IdealPVariant=Disabled  IVariant=InternalParameters  DVariant=Disabled  IntegratorVariant=Continuous  SatVariant=Disabled  AWVariant=Passthrough  PCopyVariant=Disabled  TRVariant=Disabled  FdbkBlocksVariant=Forward  IdealPFdbkVariant=Disabled  SatFdbkVariant=Disabled  DerivativeFilterVariant=Disabled  NVariant=Disabled  NCopyVariant=Disabled_SignalSpec  FilterICVariant=Disabled  IntegratorICVariant=InternalICs  ExternalResetVariant=Disabled  TRSumVariant=Passthrough  SumFdbkVariant=Disabled  SumVariant=Sum_PI  TsampFilterVariant=InternalTs  TsampNgainVariant=Passthrough  TsampIntegralVariant=Passthrough  ExternalSaturationOutDataTypeStr=Inherit: Same as second input
  PID Controller1 : pid_lib/PID Controller  Controller=PI  Form=Parallel  TimeDomain=Continuous-time  UseExternalTs=off  SampleTime=-1  IntegratorMethod=Forward Euler  FilterMethod=Forward Euler  ControllerParametersSource=internal  P=0.2  I=0.1  D=0  UseFilter=on  N=100  TunerSelectOption=Transfer Function Based (PID Tuner App)  InitialConditionSource=internal  InitialConditionForIntegrator=0  InitialConditionForFilter=0  DifferentiatorICPrevScaledInput=0  ExternalReset=none  TrackingMode=off  Kt=1  LimitOutput=off  SatLimitsSource=internal  UpperSaturationLimit=inf  LowerSaturationLimit=-inf  LinearizeAsGain=on  AntiWindupMode=none  Kb=1  POutMin=[]  POutMax=[]  IOutMin=[]  IOutMax=[]  DOutMin=[]  DOutMax=[]  NOutMin=[]  NOutMax=[]  SumOutMin=[]  SumOutMax=[]  SaturationOutMin=[]  SaturationOutMax=[]  PParamMin=[]  PParamMax=[]  IParamMin=[]  IParamMax=[]  DParamMin=[]  DParamMax=[]  NParamMin=[]  NParamMax=[]  KbParamMin=[]  KbParamMax=[]  KtParamMin=[]  KtParamMax=[]  KbOutMin=[]  KbOutMax=[]  KtOutMin=[]  KtOutMax=[]  IntegratorOutMin=[]  IntegratorOutMax=[]  FilterOutMin=[]  FilterOutMax=[]  SumI1OutMin=[]  SumI1OutMax=[]  SumI2OutMin=[]  SumI2OutMax=[]  SumI3OutMin=[]  SumI3OutMax=[]  SumI4OutMin=[]  SumI4OutMax=[]  SumDOutMin=[]  SumDOutMax=[]  DifferentiatorOutMin=[]  DifferentiatorOutMax=[]  FilterDiffOutCoefMin=[]  FilterDiffOutCoefMax=[]  ReciprocalOutMin=[]  ReciprocalOutMax=[]  SumDenOutMin=[]  SumDenOutMax=[]  SumNumOutMin=[]  SumNumOutMax=[]  DivideOutMin=[]  DivideOutMax=[]  UdiffTsProdOutMin=[]  UdiffTsProdOutMax=[]  NTsProdOutMin=[]  NTsProdOutMax=[]  UintegralTsProdOutMin=[]  UintegralTsProdOutMax=[]  UngainTsProdOutMin=[]  UngainTsProdOutMax=[]  IntegratorContinuousStateAttributes=''  IntegratorStateMustResolveToSignalObject=off  IntegratorRTWStateStorageClass=Auto  FilterContinuousStateAttributes=''  FilterStateMustResolveToSignalObject=off  FilterRTWStateStorageClass=Auto  ParallelPVariant=InternalParameters  IdealPVariant=Disabled  IVariant=InternalParameters  DVariant=Disabled  IntegratorVariant=Continuous  SatVariant=Disabled  AWVariant=Passthrough  PCopyVariant=Disabled  TRVariant=Disabled  FdbkBlocksVariant=Forward  IdealPFdbkVariant=Disabled  SatFdbkVariant=Disabled  DerivativeFilterVariant=Disabled  NVariant=Disabled  NCopyVariant=Disabled_SignalSpec  FilterICVariant=Disabled  IntegratorICVariant=InternalICs  ExternalResetVariant=Disabled  TRSumVariant=Passthrough  SumFdbkVariant=Disabled  SumVariant=Sum_PI  TsampFilterVariant=InternalTs  TsampNgainVariant=Passthrough  TsampIntegralVariant=Passthrough  ExternalSaturationOutDataTypeStr=Inherit: Same as second input
  Scope : Scope  NumInputPorts=2
  Scope1 : Scope
  Sum : Sum  Inputs=|+-
  Sum1 : Sum  Inputs=|++
  Sum2 : Sum  Inputs=|+++
  Sum3 : Sum  Inputs=|-+
  Sum4 : Sum  Inputs=|+++
  Sum5 : Sum  Inputs=|++
  Sum6 : Sum  Inputs=|++
  Vd : Outport
  Vq : Outport  Port=2
  wires:
  Id*/1 -> Multiply3/1, Derivative/1, Multiply6/1, Sum/1
  Id/1 -> Sum/2
  Derivative/1 -> Multiply/1
  Multiply/1 -> Sum1/1
  Multiply6/1 -> Sum1/2
  Sum1/1 -> Sum2/1
  PID Controller/1 -> Sum2/2
  Sum/1 -> Scope/1, PID Controller/1
  Multiply1/1 -> Sum2/3
  We/1 -> Multiply2/1
  Iq*/1 -> Multiply5/1, Derivative1/1, Sum3/2, Divide/2
  Multiply2/1 -> Divide1/2, Divide/1
  Divide/1 -> Multiply1/1
  Sum2/1 -> Scope1/1, Vd/1
  Iq/1 -> Sum3/1
  Sum3/1 -> Scope/2, PID Controller1/1
  PID Controller1/1 -> Sum4/2
  Multiply3/1 -> Sum5/1
  Constant1/1 -> Sum5/2
  Sum5/1 -> Divide1/1
  Divide1/1 -> Sum4/1
  Multiply5/1 -> Sum6/2
  Multiply4/1 -> Sum6/1
  Derivative1/1 -> Multiply4/1
  Sum6/1 -> Sum4/3
  Sum4/1 -> Vq/1

== system Model_15_11062020_3_Lev_Unbalance_SVM_AB21/3-Level NPC Inverter/Diode Loss Calculation ==
  note: Reverse Recovery Losses (W)
  note: Total Losses (W)
  note: Conduction Losses (W)
  m : Inport
  Tj_Diode : Inport  Port=2
  2-D Lookup Table_Vf_on_Diode_Pcond : Lookup_n-D  BreakpointsForDimension1=Cond_Loss_Diode.Tj  BreakpointsForDimension2=Cond_Loss_Diode.Ic  BreakpointsForDimension3=Page_Temp_C  Table=Cond_Loss_Diode.Vce  RndMeth=Simplest  InputSameDT=on
      settings: InputPortMap=u0,u1
  3-D Lookup Table_Erec_Diode : Lookup_n-D  NumberOfTableDimensions=3  BreakpointsForDimension1=Reverse_Rec_Diode.Vcc_Esw_Erec  BreakpointsForDimension2=Reverse_Rec_Diode.DIODE_If_Erec  BreakpointsForDimension3=Reverse_Rec_Diode.DIODE_Tj_Erec  Table=Reverse_Rec_Diode.Esw_Erec  RndMeth=Simplest  InputSameDT=on
      settings: InputPortMap=u0,u1,u2
  Add6 : Sum
  Bias : Bias  Bias=1e-3
  Compare To Zero4 : simulink/Logic and Bit Operations/Compare To Zero  relop===  OutDataTypeStr=boolean
  Compare To Zero5 : simulink/Logic and Bit Operations/Compare To Zero  relop=>  OutDataTypeStr=boolean
  Demux2 : Demux  Outputs=2
  Energy-to-Power 3 : Subsystem  mask{PulseDuration=PulseDuration, Ts=Ts}
      mask prompts: PulseDuration "Pulse Duration (s):"; Ts "Sample time (s):"
  Gain : Gain  Gain=1000
  Gain1 : Gain  Gain=-1
  Logical Operator2 : Logic  AllPortsSameDT=off  OutDataTypeStr=float('double')
  Mean1 : spsMeanLib/Mean  Freq=Freq  Vinit=0  Ts=0
  Mean2 : spsMeanLib/Mean  Freq=Freq  Vinit=0  Ts=0
  Memory4 : Memory
  Product3 : Product  RndMeth=Zero
  Product4 : Product  RndMeth=Zero
  Saturation4 : Saturate  UpperLimit=inf  LowerLimit=0
  Saturation5 : Saturate  UpperLimit=inf  LowerLimit=0
  Saturation6 : Saturate  UpperLimit=0  LowerLimit=-1e6
  Scope : Scope  NumInputPorts=2
  Scope1 : Scope
  Ptot : Outport  VectorParamsAs1DForOutWhenUnconnected=off
  tag scope: P_con_D1D2=global, P_switch_D1=global
  wires:
  Add6/1 -> Ptot/1
  Compare To Zero5/1 -> Logical Operator2/1
  [Diode_Tj] -> 3-D Lookup Table_Erec_Diode/3, 2-D Lookup Table_Vf_on_Diode_Pcond/1
  Product3/1 -> Saturation4/1
  Energy-to-Power 3/1(P_W) -> Saturation5/1
  Saturation5/1 -> Mean2/1, Add6/1  "Psw"
  3-D Lookup Table_Erec_Diode/1 -> Product4/2  "Erec_mJ"
  Saturation4/1 -> Add6/2, Mean1/1  "Pcond"
  Demux2/2 -> 3-D Lookup Table_Erec_Diode/1
  Memory4/1 -> 3-D Lookup Table_Erec_Diode/2, Compare To Zero5/1
  Saturation6/1 -> Gain1/1
  m/1 -> Demux2/1
  Demux2/1 -> Bias/1
  2-D Lookup Table_Vf_on_Diode_Pcond/1 -> Product3/1  "Vf_on_Diode"
  Gain1/1 -> Compare To Zero4/1, 2-D Lookup Table_Vf_on_Diode_Pcond/2, Product3/2, Memory4/1  "If"
  Logical Operator2/1 -> Gain/1, Product4/1, Energy-to-Power 3/1(Trig)
  Compare To Zero4/1 -> Logical Operator2/2
  Tj_Diode/1 -> [Diode_Tj]
  Mean1/1 -> [P_con_D1D2]
  Mean2/1 -> [P_switch_D1]
  Bias/1 -> Scope/1, Saturation6/1
  Gain/1 -> Scope/2
  Product4/1 -> Scope1/1, Energy-to-Power 3/2(E_mJ)

== system Model_15_11062020_3_Lev_Unbalance_SVM_AB21/3-Level NPC Inverter/Diode Loss Calculation1 ==
  note: Reverse Recovery Losses (W)
  note: Total Losses (W)
  note: Conduction Losses (W)
  m : Inport
  Tj_Diode : Inport  Port=2
  2-D Lookup Table_Vf_on_Diode_Pcond : Lookup_n-D  BreakpointsForDimension1=Cond_Loss_Diode.Tj  BreakpointsForDimension2=Cond_Loss_Diode.Ic  BreakpointsForDimension3=Page_Temp_C  Table=Cond_Loss_Diode.Vce  RndMeth=Simplest  InputSameDT=on
      settings: InputPortMap=u0,u1
  3-D Lookup Table_Erec_Diode : Lookup_n-D  NumberOfTableDimensions=3  BreakpointsForDimension1=Reverse_Rec_Diode.Vcc_Esw_Erec  BreakpointsForDimension2=Reverse_Rec_Diode.DIODE_If_Erec  BreakpointsForDimension3=Reverse_Rec_Diode.DIODE_Tj_Erec  Table=Reverse_Rec_Diode.Esw_Erec  RndMeth=Simplest  InputSameDT=on
      settings: InputPortMap=u0,u1,u2
  Add6 : Sum
  Bias : Bias  Bias=-1e-3
  Compare To Zero4 : simulink/Logic and Bit Operations/Compare To Zero  relop===  OutDataTypeStr=boolean
  Compare To Zero5 : simulink/Logic and Bit Operations/Compare To Zero  relop=>  OutDataTypeStr=boolean
  Demux2 : Demux  Outputs=2
  Energy-to-Power 3 : Subsystem  mask{PulseDuration=PulseDuration, Ts=Ts}
      mask prompts: PulseDuration "Pulse Duration (s):"; Ts "Sample time (s):"
  Gain1 : Gain  Gain=-1
  Logical Operator2 : Logic  AllPortsSameDT=off  OutDataTypeStr=float('double')
  Mean1 : spsMeanLib/Mean  Commented=on  Freq=50  Vinit=0  Ts=0
  Mean2 : spsMeanLib/Mean  Commented=on  Freq=50  Vinit=0  Ts=0
  Memory4 : Memory
  Product3 : Product  RndMeth=Zero
  Product4 : Product  RndMeth=Zero
  Saturation4 : Saturate  UpperLimit=inf  LowerLimit=0
  Saturation5 : Saturate  UpperLimit=inf  LowerLimit=0
  Saturation6 : Saturate  UpperLimit=0  LowerLimit=-1e6
  Scope : Scope
  Terminator : Terminator  Commented=on
  Terminator1 : Terminator  Commented=on
  Ptot : Outport  VectorParamsAs1DForOutWhenUnconnected=off
  wires:
  Add6/1 -> Ptot/1
  Compare To Zero5/1 -> Logical Operator2/1
  [Diode_Tj] -> 3-D Lookup Table_Erec_Diode/3, 2-D Lookup Table_Vf_on_Diode_Pcond/1
  Product3/1 -> Saturation4/1
  Energy-to-Power 3/1(P_W) -> Saturation5/1
  Product4/1 -> Energy-to-Power 3/2(E_mJ)
  Saturation5/1 -> Add6/1, Mean2/1  "Psw"
  3-D Lookup Table_Erec_Diode/1 -> Product4/2  "Erec_mJ"
  Saturation4/1 -> Add6/2, Mean1/1  "Pcond"
  Demux2/2 -> 3-D Lookup Table_Erec_Diode/1
  Memory4/1 -> 3-D Lookup Table_Erec_Diode/2, Compare To Zero5/1
  Saturation6/1 -> Gain1/1
  m/1 -> Demux2/1
  Demux2/1 -> Bias/1
  2-D Lookup Table_Vf_on_Diode_Pcond/1 -> Scope/1, Product3/1  "Vf_on_Diode"
  Gain1/1 -> Compare To Zero4/1, 2-D Lookup Table_Vf_on_Diode_Pcond/2, Product3/2, Memory4/1  "If"
  Logical Operator2/1 -> Product4/1, Energy-to-Power 3/1(Trig)
  Compare To Zero4/1 -> Logical Operator2/2
  Tj_Diode/1 -> [Diode_Tj]
  Mean1/1 -> Terminator1/1
  Mean2/1 -> Terminator/1
  Bias/1 -> Saturation6/1

== system Model_15_11062020_3_Lev_Unbalance_SVM_AB21/3-Level NPC Inverter/Diode Loss Calculation2 ==
  note: Reverse Recovery Losses (W)
  note: Total Losses (W)
  note: Conduction Losses (W)
  m : Inport
  Tj_Diode : Inport  Port=2
  2-D Lookup Table_Vf_on_Diode_Pcond : Lookup_n-D  BreakpointsForDimension1=Cond_Loss_Diode.Tj  BreakpointsForDimension2=Cond_Loss_Diode.Ic  BreakpointsForDimension3=Page_Temp_C  Table=Cond_Loss_Diode.Vce  RndMeth=Simplest  InputSameDT=on
      settings: InputPortMap=u0,u1
  3-D Lookup Table_Erec_Diode : Lookup_n-D  NumberOfTableDimensions=3  BreakpointsForDimension1=Reverse_Rec_Diode.Vcc_Esw_Erec  BreakpointsForDimension2=Reverse_Rec_Diode.DIODE_If_Erec  BreakpointsForDimension3=Reverse_Rec_Diode.DIODE_Tj_Erec  Table=Reverse_Rec_Diode.Esw_Erec  RndMeth=Simplest  InputSameDT=on
      settings: InputPortMap=u0,u1,u2
  Add6 : Sum
  Bias : Bias  Bias=1e-3
  Compare To Zero4 : simulink/Logic and Bit Operations/Compare To Zero  relop===  OutDataTypeStr=boolean
  Compare To Zero5 : simulink/Logic and Bit Operations/Compare To Zero  relop=>  OutDataTypeStr=boolean
  Demux2 : Demux  Outputs=2
  Energy-to-Power 3 : Subsystem  mask{PulseDuration=PulseDuration, Ts=Ts}
      mask prompts: PulseDuration "Pulse Duration (s):"; Ts "Sample time (s):"
  Gain : Gain  Gain=1000
  Gain1 : Gain  Gain=-1
  Logical Operator2 : Logic  AllPortsSameDT=off  OutDataTypeStr=float('double')
  Mean1 : spsMeanLib/Mean  Freq=Freq  Vinit=0  Ts=0
  Mean2 : spsMeanLib/Mean  Freq=Freq  Vinit=0  Ts=0
  Memory4 : Memory
  Product3 : Product  RndMeth=Zero
  Product4 : Product  RndMeth=Zero
  Saturation4 : Saturate  UpperLimit=inf  LowerLimit=0
  Saturation5 : Saturate  UpperLimit=inf  LowerLimit=0
  Saturation6 : Saturate  UpperLimit=0  LowerLimit=-1e6
  Scope : Scope  NumInputPorts=2
  Scope1 : Scope
  Ptot : Outport  VectorParamsAs1DForOutWhenUnconnected=off
  tag scope: P_con_D3=global, P_switch_D3=global
  wires:
  Add6/1 -> Ptot/1
  Compare To Zero5/1 -> Logical Operator2/1
  [Diode_Tj] -> 3-D Lookup Table_Erec_Diode/3, 2-D Lookup Table_Vf_on_Diode_Pcond/1
  Product3/1 -> Saturation4/1
  Energy-to-Power 3/1(P_W) -> Saturation5/1
  Saturation5/1 -> Mean2/1, Add6/1  "Psw"
  3-D Lookup Table_Erec_Diode/1 -> Product4/2  "Erec_mJ"
  Saturation4/1 -> Add6/2, Mean1/1  "Pcond"
  Demux2/2 -> 3-D Lookup Table_Erec_Diode/1
  Memory4/1 -> 3-D Lookup Table_Erec_Diode/2, Compare To Zero5/1
  Saturation6/1 -> Gain1/1
  m/1 -> Demux2/1
  Demux2/1 -> Bias/1
  2-D Lookup Table_Vf_on_Diode_Pcond/1 -> Product3/1  "Vf_on_Diode"
  Gain1/1 -> Compare To Zero4/1, 2-D Lookup Table_Vf_on_Diode_Pcond/2, Product3/2, Memory4/1  "If"
  Logical Operator2/1 -> Gain/1, Product4/1, Energy-to-Power 3/1(Trig)
  Compare To Zero4/1 -> Logical Operator2/2
  Tj_Diode/1 -> [Diode_Tj]
  Mean1/1 -> [P_con_D3]
  Mean2/1 -> [P_switch_D3]
  Bias/1 -> Scope/1, Saturation6/1
  Gain/1 -> Scope/2
  Product4/1 -> Scope1/1, Energy-to-Power 3/2(E_mJ)

== system Model_15_11062020_3_Lev_Unbalance_SVM_AB21/3-Level NPC Inverter/Diode Loss Calculation3 ==
  note: Reverse Recovery Losses (W)
  note: Total Losses (W)
  note: Conduction Losses (W)
  m : Inport
  Tj_Diode : Inport  Port=2
  2-D Lookup Table_Vf_on_Diode_Pcond : Lookup_n-D  BreakpointsForDimension1=Cond_Loss_Diode.Tj  BreakpointsForDimension2=Cond_Loss_Diode.Ic  BreakpointsForDimension3=Page_Temp_C  Table=Cond_Loss_Diode.Vce  RndMeth=Simplest  InputSameDT=on
      settings: InputPortMap=u0,u1
  3-D Lookup Table_Erec_Diode : Lookup_n-D  NumberOfTableDimensions=3  BreakpointsForDimension1=Reverse_Rec_Diode.Vcc_Esw_Erec  BreakpointsForDimension2=Reverse_Rec_Diode.DIODE_If_Erec  BreakpointsForDimension3=Reverse_Rec_Diode.DIODE_Tj_Erec  Table=Reverse_Rec_Diode.Esw_Erec  RndMeth=Simplest  InputSameDT=on
      settings: InputPortMap=u0,u1,u2
  Add6 : Sum
  Bias : Bias  Bias=-1e-3
  Compare To Zero4 : simulink/Logic and Bit Operations/Compare To Zero  relop===  OutDataTypeStr=boolean
  Compare To Zero5 : simulink/Logic and Bit Operations/Compare To Zero  relop=>  OutDataTypeStr=boolean
  Demux2 : Demux  Outputs=2
  Energy-to-Power 3 : Subsystem  mask{PulseDuration=PulseDuration, Ts=Ts}
      mask prompts: PulseDuration "Pulse Duration (s):"; Ts "Sample time (s):"
  Gain1 : Gain  Gain=-1
  Logical Operator2 : Logic  AllPortsSameDT=off  OutDataTypeStr=float('double')
  Mean1 : spsMeanLib/Mean  Commented=on  Freq=50  Vinit=0  Ts=0
  Mean2 : spsMeanLib/Mean  Commented=on  Freq=50  Vinit=0  Ts=0
  Memory4 : Memory
  Product3 : Product  RndMeth=Zero
  Product4 : Product  RndMeth=Zero
  Saturation4 : Saturate  UpperLimit=inf  LowerLimit=0
  Saturation5 : Saturate  UpperLimit=inf  LowerLimit=0
  Saturation6 : Saturate  UpperLimit=0  LowerLimit=-1e6
  Scope : Scope
  Terminator : Terminator  Commented=on
  Terminator1 : Terminator  Commented=on
  Ptot : Outport  VectorParamsAs1DForOutWhenUnconnected=off
  wires:
  Add6/1 -> Ptot/1
  Compare To Zero5/1 -> Logical Operator2/1
  [Diode_Tj] -> 3-D Lookup Table_Erec_Diode/3, 2-D Lookup Table_Vf_on_Diode_Pcond/1
  Product3/1 -> Saturation4/1
  Energy-to-Power 3/1(P_W) -> Saturation5/1
  Product4/1 -> Energy-to-Power 3/2(E_mJ)
  Saturation5/1 -> Add6/1, Mean2/1  "Psw"
  3-D Lookup Table_Erec_Diode/1 -> Product4/2  "Erec_mJ"
  Saturation4/1 -> Add6/2, Mean1/1  "Pcond"
  Demux2/2 -> 3-D Lookup Table_Erec_Diode/1
  Memory4/1 -> 3-D Lookup Table_Erec_Diode/2, Compare To Zero5/1
  Saturation6/1 -> Gain1/1
  m/1 -> Demux2/1
  Demux2/1 -> Bias/1
  2-D Lookup Table_Vf_on_Diode_Pcond/1 -> Scope/1, Product3/1  "Vf_on_Diode"
  Gain1/1 -> Compare To Zero4/1, 2-D Lookup Table_Vf_on_Diode_Pcond/2, Product3/2, Memory4/1  "If"
  Logical Operator2/1 -> Product4/1, Energy-to-Power 3/1(Trig)
  Compare To Zero4/1 -> Logical Operator2/2
  Tj_Diode/1 -> [Diode_Tj]
  Mean1/1 -> Terminator1/1
  Mean2/1 -> Terminator/1
  Bias/1 -> Saturation6/1

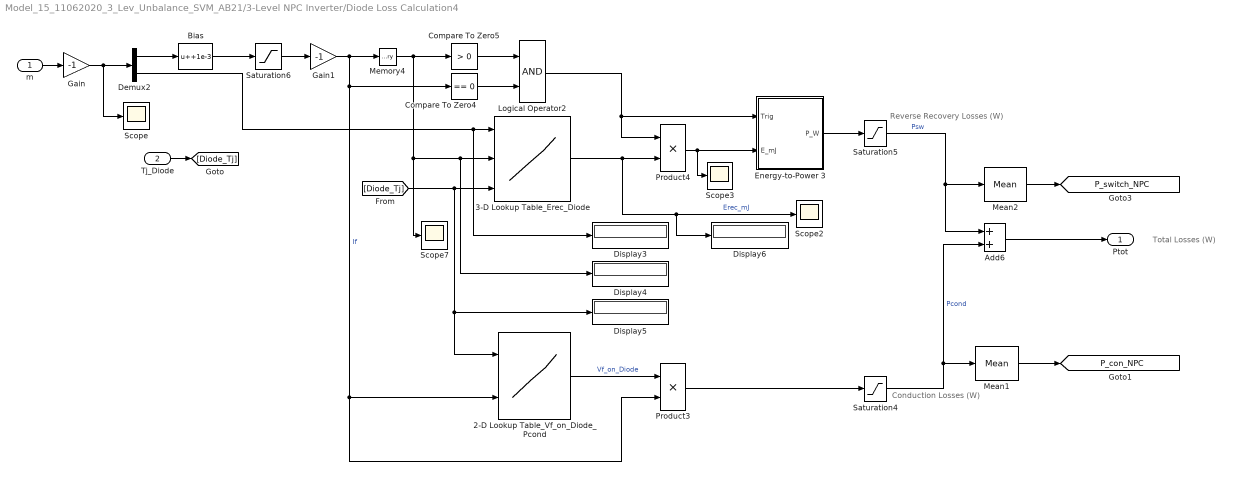
== system Model_15_11062020_3_Lev_Unbalance_SVM_AB21/3-Level NPC Inverter/Diode Loss Calculation4 ==
  note: Conduction Losses (W)
  note: Total Losses (W)
  note: Reverse Recovery Losses (W)
  m : Inport
  Tj_Diode : Inport  Port=2
  2-D Lookup Table_Vf_on_Diode_Pcond : Lookup_n-D  BreakpointsForDimension1=Cond_Loss_Diode.Tj  BreakpointsForDimension2=Cond_Loss_Diode.Ic  BreakpointsForDimension3=Page_Temp_C  Table=Cond_Loss_Diode.Vce  RndMeth=Simplest  InputSameDT=on
      settings: InputPortMap=u0,u1
  3-D Lookup Table_Erec_Diode : Lookup_n-D  NumberOfTableDimensions=3  BreakpointsForDimension1=Reverse_Rec_Diode.Vcc_Esw_Erec  BreakpointsForDimension2=Reverse_Rec_Diode.DIODE_If_Erec  BreakpointsForDimension3=Reverse_Rec_Diode.DIODE_Tj_Erec  Table=Reverse_Rec_Diode.Esw_Erec  RndMeth=Simplest  InputSameDT=on
      settings: InputPortMap=u0,u1,u2
  Add6 : Sum
  Bias : Bias  Bias=+1e-3
  Compare To Zero4 : simulink/Logic and Bit Operations/Compare To Zero  relop===  OutDataTypeStr=boolean
  Compare To Zero5 : simulink/Logic and Bit Operations/Compare To Zero  relop=>  OutDataTypeStr=boolean
  Demux2 : Demux  Outputs=2
  Display{3..6} (4 alike) : Display
  Energy-to-Power 3 : Subsystem  mask{PulseDuration=PulseDuration, Ts=Ts}
      mask prompts: PulseDuration "Pulse Duration (s):"; Ts "Sample time (s):"
  Gain : Gain  Gain=-1
  Gain1 : Gain  Gain=-1
  Logical Operator2 : Logic  AllPortsSameDT=off  OutDataTypeStr=float('double')
  Mean1 : spsMeanLib/Mean  Freq=Freq  Vinit=0  Ts=0
  Mean2 : spsMeanLib/Mean  Freq=Freq  Vinit=0  Ts=0
  Memory4 : Memory
  Product3 : Product  RndMeth=Zero
  Product4 : Product  RndMeth=Zero
  Saturation4 : Saturate  UpperLimit=inf  LowerLimit=0
  Saturation5 : Saturate  UpperLimit=inf  LowerLimit=0
  Saturation6 : Saturate  UpperLimit=0  LowerLimit=-1e6
  Scope{,2..3,7} (4 alike) : Scope
  Ptot : Outport  VectorParamsAs1DForOutWhenUnconnected=off
  tag scope: P_con_NPC=global, P_switch_NPC=global
  wires:
  Tj_Diode/1 -> [Diode_Tj]
  Compare To Zero4/1 -> Logical Operator2/2
  Logical Operator2/1 -> Energy-to-Power 3/1(Trig), Product4/1
  Gain1/1 -> Memory4/1, Product3/2, 2-D Lookup Table_Vf_on_Diode_Pcond/2, Compare To Zero4/1  "If"
  2-D Lookup Table_Vf_on_Diode_Pcond/1 -> Product3/1  "Vf_on_Diode"
  Demux2/1 -> Bias/1
  m/1 -> Gain/1
  Saturation6/1 -> Gain1/1
  Memory4/1 -> Compare To Zero5/1, Scope7/1, Display4/1, 3-D Lookup Table_Erec_Diode/2
  Demux2/2 -> Display3/1, 3-D Lookup Table_Erec_Diode/1
  Saturation4/1 -> Mean1/1, Add6/2  "Pcond"
  3-D Lookup Table_Erec_Diode/1 -> Display6/1, Scope2/1, Product4/2  "Erec_mJ"
  Saturation5/1 -> Mean2/1, Add6/1  "Psw"
  Product4/1 -> Scope3/1, Energy-to-Power 3/2(E_mJ)
  Energy-to-Power 3/1(P_W) -> Saturation5/1
  Product3/1 -> Saturation4/1
  [Diode_Tj] -> Display5/1, 2-D Lookup Table_Vf_on_Diode_Pcond/1, 3-D Lookup Table_Erec_Diode/3
  Compare To Zero5/1 -> Logical Operator2/1
  Add6/1 -> Ptot/1
  Bias/1 -> Saturation6/1
  Gain/1 -> Scope/1, Demux2/1
  Mean2/1 -> [P_switch_NPC]
  Mean1/1 -> [P_con_NPC]
